simulink model "controladorModelo"  (Simulink 8.1)
settings: Solver=ode45  StartTime=0.0  StopTime=45  RelTol=1e-3
undefined symbols (not defined in the file): sigbuilder_block
libraries: fuzblock x1
settings Model: Creator=alunoccc  LastModifiedBy=Samara
settings DebuggingCC: StrictBusMsg=Warning

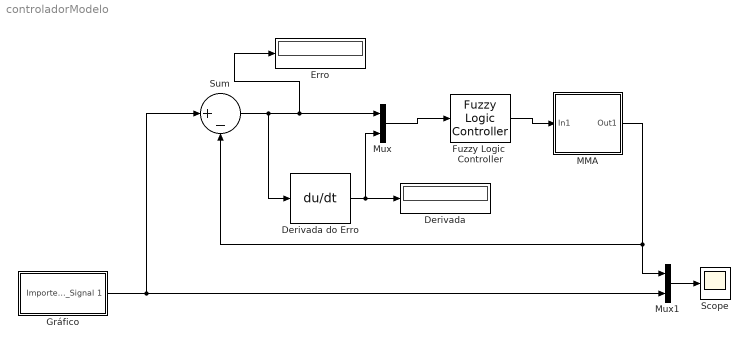
== system controladorModelo ==
  Derivada : Display
  Derivada do Erro : Derivative
  Erro : Display
  Fuzzy Logic  Controller : fuzblock/Fuzzy Logic  Controller  fis='controladorfuzzy.fis'
  Gráfico : Subsystem  Tag=STV Subsys  LoadFcn=sigbuilder_block('load');  StartFcn=sigbuilder_block('start');  StopFcn=sigbuilder_block('stop');  ClipboardFcn=sigbuilder_block('clipboard');  mask(Sigbuilder block){}
      mask help: Simulink:masks:SigbuilderBlock_MD
      mask init:
      | if ~strcmp(get_param(bdroot(gcbh),'SimulationStatus'),'stopped') tuvar = sigbuilder_block('maskInit'); end
      settings: CopyFcn=sigbuilder_block('copy');  DeleteFcn=sigbuilder_block('delete');  ModelCloseFcn=sigbuilder_block('modelClose');  PreSaveFcn=sigbuilder_block('preSave');  PauseFcn=sigbuilder_block('pause');  ContinueFcn=sigbuilder_block('continue');  NameChangeFcn=sigbuilder_block('namechange');  OpenFcn=sigbuilder_block('open',[518.25 36 500.25 477 ]);  CloseFcn=sigbuilder_block('close');
      mask Display: plot(0, 0, 100, 100,[2, 2, 32, 32, 2], [68, 8, 8, 68, 68],[32, 2], [38, 38], [32, 19, 2],[53, 60, 44], [32, 17, 17, 2],[16, 16, 31, 31]);txt = getActiveGroup(gcbh);text(2, 100, txt,'verticalAlignment', 'top');
  MMA : Subsystem
  Mux : Mux  Inputs=2
  Mux1 : Mux  Inputs=2
  Scope : Scope
      settings: TickLabels=on  TimeRange=45  YMin=0  YMax=2.1  SampleInput=on
  Sum : Sum  Inputs=|+-
  wires:
  Sum/1 -> Erro/1, Mux/1, Derivada do Erro/1
  Derivada do Erro/1 -> Derivada/1, Mux/2
  Gráfico/1(Imported_Signal 1) -> Sum/1, Mux1/2
  MMA/1(Out1) -> Mux1/1, Sum/2
  Mux1/1 -> Scope/1
  Mux/1 -> Fuzzy Logic  Controller/1
  Fuzzy Logic  Controller/1 -> MMA/1(In1)

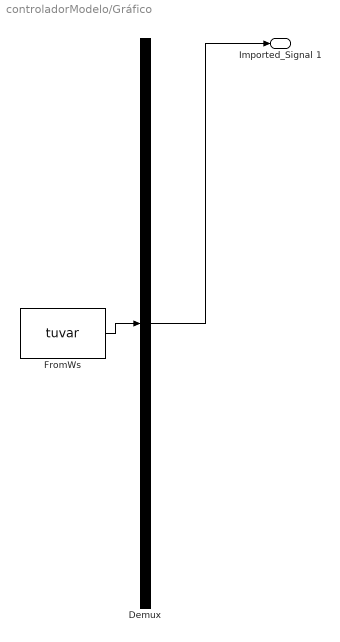
== system controladorModelo/Gráfico ==
  Demux : Demux  Tag=STV Demux  Outputs=1
  FromWs : FromWorkspace  Tag=STV FromWs  VariableName=tuvar  SampleTime=0  SigBuilderData=DataTag0  VnvData=DataTag1
      SigBuilderData=|
      | common.afterFinalStr = 'Extrapolate'
      | common.sampleTime = 0
      | dataSet.timeRange = [0 45]
      | dataSet.name = 'Plan1'
      | sbobj.Name = 'Signal Builder'
      | sbobj.Groups.Name = 'Plan1'
      | sbobj.Groups.Signals.Name = 'Imported_Signal 1'
      | sbobj.Groups.Signals.XData = [0 3 3 15 21 30 30 45]
      | sbobj.Groups.Signals.YData = [0 0 1 1 2 2 0.5 0.5]
      | sbobj.Groups.TimeRange = [0 45]
  Imported_Signal 1 : Outport
  wires:
  Demux/1 -> Imported_Signal 1/1
  FromWs/1 -> Demux/1

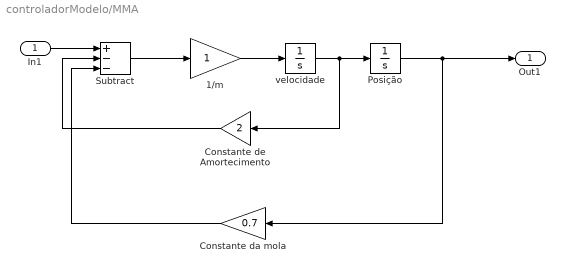
== system controladorModelo/MMA ==
  In1 : Inport
  1/m : Gain
  Constante da mola : Gain  Gain=0.7
  Constante de Amortecimento : Gain  Gain=2
  Posição : Integrator
  Subtract : Sum  Inputs=+--
  velocidade : Integrator
  Out1 : Outport
  wires:
  velocidade/1 -> Constante de Amortecimento/1, Posição/1
  1/m/1 -> velocidade/1
  Subtract/1 -> 1/m/1
  In1/1 -> Subtract/1
  Constante de Amortecimento/1 -> Subtract/2
  Constante da mola/1 -> Subtract/3
  Posição/1 -> Constante da mola/1, Out1/1
